simulink model "main_RI_LIEKF"  (R2023a)
settings: Solver=FixedStepAuto  StartTime=0.0  StopTime=220  FixedStep=0.01  RelTol=1e-3
InitFcn:
  | initNavigation0612_AOA;
values from neighbouring files (symbols this model uses):
  CF_enable = 0    [initNavigation.m]
  dt = 0.01    [initNavigation.m]
  dtDelay = -0.03    [initNavigation.m]
  g0 = 9.795    [initNavigation.m]
  gam0_rad = 0/57.3    (= 0)    [initNavigation.m]
  H_sensor_type = 0    [initNavigation.m]
  KF_enable = 1    [initNavigation.m]
  P0 = diag([1*ones(3,1);0.01*ones(3,1);0.1*ones(3,1);0.001*ones(3,1);0.00001*ones(3,1)])    [initNavigation.m]
  P0_RIEKF = diag([1*ones(3,1);0.01*ones(3,1);0.1*ones(3,1);0.001*ones(3,1);0.00001*ones(3,1);      0.01*ones(3,1);[0;2;2]/57.3;[0.1;0.1;0.1]])^2    [initNavigation.m]
  pd0 = 0    [initNavigation.m]
  pe0 = 0    [initNavigation.m]
  phi0_rad = 0/57.3    (= 0)    [initNavigation.m]
  pn0 = 0    [initNavigation.m]
  psi = -178    [initNavigation.m]
  psi0_rad = 0/57.3    (= 0)    [initNavigation.m]
  state_dim = 24    [initNavigation.m]
  Time = 0:0.01:(size(traindata.AttackAngle,1) - 1)*0.01    [NNLiftCoefficientFit.m]
  vd0 = 0    [initNavigation.m]
  ve0 = 0    [initNavigation.m]
  vn0 = 0    [initNavigation.m]
undefined symbols (not defined in the file or in its folder): DiscIntNeverNeededParam, Discrete, INS_CONST, INS_EXPORT, INS_PARAM, magnitude, p, param, pInitialization, sys
libraries: simulink x69, simulink_extras x64, dspstat3 x56, sharedtransform x49, ctrlSharedLib x36, sharedTrackingLibrary x17, FMT_Model_Lib x13, matrix_library x12, deeplib x4, dspsolvers x4, vrlib x4, aerolibconvert2 x1
(part 17 of 22)

== system main_RI_LIEKF/State estimation/distribute CF/distribute CF/Correct/Attitude_Correction/Attitude_Correct ==
  Sensor_Data : Inport
  Rotation_Data : Inport  Port=2
  Acc_Correct : Subsystem
  Subsystem2 : Subsystem
  att_corr_O : Outport
  wires:
  Subsystem2/2(acc_meas_O_mPs2) -> Acc_Correct/2(acc_meas_O_mPs2)  "GPS-加速度估计"
  Acc_Correct/1(att_correct) -> att_corr_O/1
  Subsystem2/3(acc_est_O_mPs2) -> Acc_Correct/3(acc_est_O_mPs2)  "加计-加速度"
  Subsystem2/1(acc_meas_valid) -> Acc_Correct/1(acc_meas_valid)  "GPS状态判断"
  Sensor_Data/1 -> Subsystem2/1(Sensor_Data)
  Rotation_Data/1 -> Subsystem2/2(Rotation_Data)

== system main_RI_LIEKF/State estimation/distribute CF/distribute CF/Correct/Attitude_Correction/Mag_Correct ==
  Rotation_Data : Inport
  Sensor_Data : Inport  Port=2
  Bus Selector1 : BusSelector  OutputSignals=MAGN_Data.mag_norm_B,MAGN_Data.mag_quality
  Bus Selector4 : BusSelector  OutputSignals=M_OB
  MX Product3 : Product  Inputs=3  RndMeth=Simplest
  MX Product4 : Product  Multiplication=Matrix(*)  RndMeth=Simplest
  Relay1 : Relay  OnSwitchValue=0.3  OffSwitchValue=0.2
  Selector4 : Selector  NumberOfDimensions=2  InputPortWidth=3  IndexOptions=Index vector (dialog),Index vector (dialog)  Indices=[2],[1 2 3]  OutputSizes=1,1
  Z axis : Constant  Value=[0 0 1]  OutDataTypeStr=single
  mag_correct_gain : Gain  Gain=MAG_GAIN  OutDataTypeStr=Inherit: Same as input
  mag_corr_O : Outport  VectorParamsAs1DForOutWhenUnconnected=off
  wires:
  Bus Selector4/1 -> Selector4/1  "<M_OB>"
  Rotation_Data/1 -> Bus Selector4/1
  Bus Selector1/2 -> Relay1/1  "<mag_quality>"
  Sensor_Data/1 -> Bus Selector1/1
  mag_correct_gain/1 -> MX Product3/2
  MX Product4/1 -> mag_correct_gain/1  "my_O"
  Selector4/1 -> MX Product4/1
  Relay1/1 -> MX Product3/3  "mag_enable"
  MX Product3/1 -> mag_corr_O/1
  Bus Selector1/1 -> MX Product4/2  "<mag_norm_B>"
  Z axis/1 -> MX Product3/1

== system main_RI_LIEKF/State estimation/distribute CF/distribute CF/Correct/Subsystem2/norm ==
  In1 : Inport
  Sqrt : Sqrt
  Square : Math  Operator=square  SignedPower=on
  Sum of Elements : Sum  Inputs=+
  Out1 : Outport
  wires:
  Sum of Elements/1 -> Sqrt/1
  Square/1 -> Sum of Elements/1
  Sqrt/1 -> Out1/1
  In1/1 -> Square/1

== system main_RI_LIEKF/State estimation/distribute CF/distribute CF/Correct/Subsystem2/低通滤波 ==
  u : Inport
  Constant : Constant  Value=0
  Discrete-Time Integrator : DiscreteIntegrator  ExternalReset=level  SampleTime=-1  ICPrevOutput=DiscIntNeverNeededParam  ICPrevScaledInput=DiscIntNeverNeededParam
  Discrete-Time Integrator1 : DiscreteIntegrator  ExternalReset=level  InitialConditionSource=external  SampleTime=-1  ICPrevOutput=DiscIntNeverNeededParam  ICPrevScaledInput=DiscIntNeverNeededParam
  Gain : Gain  Gain=(2*pi*fc)^2
  Gain1 : Gain  Gain=2*zeta*(2*pi*fc)
  Sum : Sum  Inputs=|+-
  Sum1 : Sum  Inputs=|+-
  y : Outport
  wires:
  Sum/1 -> Gain/1
  Discrete-Time Integrator1/1 -> y/1, Sum/2
  Discrete-Time Integrator/1 -> Gain1/1, Discrete-Time Integrator1/1
  Sum1/1 -> Discrete-Time Integrator/1
  Constant/1 -> Discrete-Time Integrator1/2, Discrete-Time Integrator/2
  u/1 -> Discrete-Time Integrator1/3, Sum/1
  Gain1/1 -> Sum1/2
  Gain/1 -> Sum1/1

== system main_RI_LIEKF/State estimation/distribute CF/distribute CF/Translation_estimate/Rxy_Horizontal_estimation/Integrator_R_Horizontal ==
  Vn : Inport
  dR : Inport  Port=2
  Sensor_data2 : Inport  Port=3
  Cbn : Inport  Port=4
  Add : Sum
  Bus Selector : BusSelector  OutputSignals=QGC_sensor_reinit,GPS_Data.pos_N_gps,GPS_Data.pos_E_gps
  Constant : Constant  Value=[-0.45;0;0]  OutDataTypeStr=single
  Delay : Delay  DelayLength=1  InitialConditionSource=Input port  ExternalReset=Rising
      settings: InputPortMap=u0,r5,p4
  Gain : Gain  Gain=0.1
  Gain2 : Gain  Gain=dt  SaturateOnIntegerOverflow=on  OutDataTypeStr=Inherit: Same as input  ParamDataTypeStr=Inherit: Same as input
  Mux : Mux  Inputs=2
  Product : Product  Multiplication=Matrix(*)
  Selector : Selector  InputPortWidth=3  IndexOptions=Index vector (dialog)  Indices=[1 2]  OutputSizes=1
  Sum : Sum  Inputs=|++-
  R_n&e : Outport
  R_n&eL : Outport  Port=2
  wires:
  dR/1 -> Gain/1
  Vn/1 -> Gain2/1
  Gain2/1 -> Sum/1
  Sensor_data2/1 -> Bus Selector/1
  Bus Selector/1 -> Delay/2  "<QGC_sensor_reinit>"
  Bus Selector/2 -> Mux/1  "<pos_N_gps>"
  Bus Selector/3 -> Mux/2  "<pos_E_gps>"
  Mux/1 -> Delay/3
  Delay/1 -> Sum/2
  Gain/1 -> Sum/3
  Constant/1 -> Product/2
  Product/1 -> Selector/1
  Cbn/1 -> Product/1
  Sum/1 -> Add/1, R_n&e/1, Delay/1
  Selector/1 -> Add/2
  Add/1 -> R_n&eL/1

== system main_RI_LIEKF/State estimation/distribute CF/distribute CF/Translation_estimate/Rxy_Horizontal_estimation/Rxy_kalman filter2 ==
  X : Inport
  Z : Inport  Port=2
  Enable : Inport  Port=3
  Constant : Constant  Value=F  OutDataTypeStr=single
  Constant1 : Constant  Value=Q  OutDataTypeStr=single
  Constant2 : Constant  Value=R  OutDataTypeStr=single
  Constant3 : Constant  Value=P0  OutDataTypeStr=single
  Constant4 : Constant  Value=H  OutDataTypeStr=single
  Vxy kalman filter : Subsystem  TreatAsAtomicUnit=on
  XOut : Outport
  wires:
  Enable/1 -> Vxy kalman filter/9(Enable)
  Vxy kalman filter/1(XOut) -> XOut/1
  Constant1/1 -> Vxy kalman filter/5(Q)
  Constant4/1 -> Vxy kalman filter/4(H)
  Constant2/1 -> Vxy kalman filter/6(R)
  Constant3/1 -> Vxy kalman filter/8(P0)
  Z/1 -> Vxy kalman filter/1(Z)
  Constant/1 -> Vxy kalman filter/3(G), Vxy kalman filter/2(F)
  X/1 -> Vxy kalman filter/7(X)

== system main_RI_LIEKF/State estimation/distribute CF/distribute CF/Translation_estimate/Rxy_Horizontal_estimation/Subsystem ==
  Detect Change1 : simulink/Logic and Bit Operations/Detect Change  vinit=0  InputProcessing=Columns as channels (frame based)  OutDataTypeStr=boolean
  From Workspace1 : FromWorkspace  VariableName=[All.t',All.lat]
  flag : Outport
  wires:
  Detect Change1/1 -> flag/1
  From Workspace1/1 -> Detect Change1/1  "lat"

== system main_RI_LIEKF/State estimation/distribute CF/distribute CF/Translation_estimate/V_Horizontal_estimation/Integrator_V_Horizontal ==
  An : Inport
  dv : Inport  Port=2
  Sensor_data2 : Inport  Port=3
  Bus Selector : BusSelector  OutputSignals=QGC_sensor_reinit,GPS_Data.vn_gps,GPS_Data.ve_gps
  Delay : Delay  DelayLength=1  InitialConditionSource=Input port  ExternalReset=Rising
      settings: InputPortMap=u0,r5,p4
  Gain : Gain
  Gain2 : Gain  Gain=dt  SaturateOnIntegerOverflow=on  OutDataTypeStr=Inherit: Same as input  ParamDataTypeStr=Inherit: Same as input
  Mux : Mux  Inputs=2
  Scope : Scope
  Sum : Sum  Inputs=|++-
  V_n&e : Outport
  wires:
  Gain/1 -> Sum/3, Scope/1
  dv/1 -> Gain/1
  Delay/1 -> Sum/2
  Mux/1 -> Delay/3
  Bus Selector/3 -> Mux/2  "<ve_gps>"
  Bus Selector/2 -> Mux/1  "<vn_gps>"
  Bus Selector/1 -> Delay/2  "<QGC_sensor_reinit>"
  Sensor_data2/1 -> Bus Selector/1
  Sum/1 -> Delay/1, V_n&e/1
  Gain2/1 -> Sum/1
  An/1 -> Gain2/1

== system main_RI_LIEKF/State estimation/distribute CF/distribute CF/Translation_estimate/V_Horizontal_estimation/Rxy_kalman filter1 ==
  X : Inport
  Z : Inport  Port=2
  Enable : Inport  Port=3
  Constant : Constant  Value=F  OutDataTypeStr=single
  Constant1 : Constant  Value=Q  OutDataTypeStr=single
  Constant2 : Constant  Value=R  OutDataTypeStr=single
  Constant3 : Constant  Value=P0  OutDataTypeStr=single
  Constant4 : Constant  Value=H  OutDataTypeStr=single
  Vxy kalman filter : Subsystem  TreatAsAtomicUnit=on
  XOut : Outport
  wires:
  X/1 -> Vxy kalman filter/7(X)
  Constant/1 -> Vxy kalman filter/2(F), Vxy kalman filter/3(G)
  Z/1 -> Vxy kalman filter/1(Z)
  Constant3/1 -> Vxy kalman filter/8(P0)
  Constant2/1 -> Vxy kalman filter/6(R)
  Constant4/1 -> Vxy kalman filter/4(H)
  Constant1/1 -> Vxy kalman filter/5(Q)
  Vxy kalman filter/1(XOut) -> XOut/1
  Enable/1 -> Vxy kalman filter/9(Enable)

== system main_RI_LIEKF/State estimation/distribute CF/distribute CF/Update/Attitude_Update/uniformization1 ==
  Q i : Inport  PortDimensions=4
  Constant : Constant  Value=1e-20
  Dot Product1 : DotProduct  OutDataTypeStr=Inherit: Inherit via internal rule
  Math Function : Math  Operator=sqrt  SignedPower=on
  Product : Product  Inputs=*/  SaturateOnIntegerOverflow=on  OutDataTypeStr=Inherit: Same as first input
  Sum : Sum  Inputs=|++  SaturateOnIntegerOverflow=on
  Q o : Outport
  wires:
  Sum/1 -> Product/2
  Constant/1 -> Sum/2
  Product/1 -> Q o/1
  Math Function/1 -> Sum/1
  Dot Product1/1 -> Math Function/1
  Q i/1 -> Product/1, Dot Product1/1, Dot Product1/2

== system main_RI_LIEKF/State estimation/distribute CF/distribute CF/初始化/Attitude_Reset/Reset Heading ==
  note: When GPS is valid at first time, the mag data will be compensated with WMM data,
      | so we need reset attitude.
  GPS_valid : Inport
  Add : Sum  AccumDataTypeStr=uint32
  Compare To Constant : simulink/Logic and Bit Operations/Compare To Constant  relop=>=  const=1  OutDataTypeStr=boolean
  Data Type Conversion : DataTypeConversion  OutDataTypeStr=uint32  SaturateOnIntegerOverflow=off  RndMeth=Floor
  Delay : Delay  DelayLength=1
  Detect Rise Positive1 : simulink/Logic and Bit Operations/Detect Rise Positive  vinit=0  OutDataTypeStr=boolean
  Saturation : Saturate  UpperLimit=1  LowerLimit=0
  reset : Outport
  wires:
  Delay/1 -> Add/2
  Data Type Conversion/1 -> Add/1
  GPS_valid/1 -> Compare To Constant/1
  Detect Rise Positive1/1 -> reset/1
  Add/1 -> Saturation/1
  Saturation/1 -> Detect Rise Positive1/1, Delay/1
  Compare To Constant/1 -> Data Type Conversion/1

== system main_RI_LIEKF/State estimation/distribute CF/distribute CF/初始化/Attitude_Reset/norm ==
  In1 : Inport
  Sqrt : Sqrt
  Square : Math  Operator=square  SignedPower=on
  Sum of Elements : Sum  Inputs=+
  Out1 : Outport
  wires:
  Sum of Elements/1 -> Sqrt/1
  Square/1 -> Sum of Elements/1
  Sqrt/1 -> Out1/1
  In1/1 -> Square/1

== system main_RI_LIEKF/State estimation/distribute CF/distribute CF/初始化/Attitude_Reset/sample_valid ==
  valid : Inport
  Add : Sum  AccumDataTypeStr=uint32
  Data Type Conversion : DataTypeConversion  OutDataTypeStr=uint32  SaturateOnIntegerOverflow=off  RndMeth=Floor
  Delay : Delay  DelayLength=1
  Saturation : Saturate  UpperLimit=10000  LowerLimit=0
  valid_samples : simulink/Logic and Bit Operations/Compare To Constant  relop=>  const=50  OutDataTypeStr=boolean
  sample_valid : Outport
  wires:
  Add/1 -> Saturation/1
  valid_samples/1 -> sample_valid/1
  Delay/1 -> Add/2
  valid/1 -> Data Type Conversion/1
  Data Type Conversion/1 -> Add/1
  Saturation/1 -> valid_samples/1, Delay/1

== system main_RI_LIEKF/State estimation/distribute CF/distribute CF/初始化/Subsystem/Normalized1 ==
  fb : Inport
  Add : Sum
  Constant : Constant  Value=1e-6  OutDataTypeStr=single
  Divide : Product  Inputs=*/
  Math Function : Math  Operator=magnitude^2  SignedPower=on
  Sqrt : Sqrt
  Sum of Elements : Sum  Inputs=+
  fb/g : Outport
  wires:
  Math Function/1 -> Sum of Elements/1
  Divide/1 -> fb/g/1
  Sum of Elements/1 -> Sqrt/1
  fb/1 -> Divide/1, Math Function/1
  Add/1 -> Divide/2
  Sqrt/1 -> Add/1
  Constant/1 -> Add/2

== system main_RI_LIEKF/State estimation/distribute CF/distribute CF/初始化/Subsystem/Normalized2 ==
  fb : Inport
  Add : Sum
  Constant : Constant  Value=1e-6  OutDataTypeStr=single
  Divide : Product  Inputs=*/
  Math Function : Math  Operator=magnitude^2  SignedPower=on
  Sqrt : Sqrt
  Sum of Elements : Sum  Inputs=+
  fb/g : Outport
  wires:
  Math Function/1 -> Sum of Elements/1
  Divide/1 -> fb/g/1
  Sum of Elements/1 -> Sqrt/1
  fb/1 -> Divide/1, Math Function/1
  Add/1 -> Divide/2
  Sqrt/1 -> Add/1
  Constant/1 -> Add/2

== system main_RI_LIEKF/State estimation/distribute CF/distribute CF/初始化/Subsystem/Normalized3 ==
  fb : Inport
  Add : Sum
  Constant : Constant  Value=1e-6  OutDataTypeStr=single
  Divide : Product  Inputs=*/
  Math Function : Math  Operator=magnitude^2  SignedPower=on
  Sqrt : Sqrt
  Sum of Elements : Sum  Inputs=+
  fb/g : Outport
  wires:
  Math Function/1 -> Sum of Elements/1
  Divide/1 -> fb/g/1
  Sum of Elements/1 -> Sqrt/1
  fb/1 -> Divide/1, Math Function/1
  Add/1 -> Divide/2
  Sqrt/1 -> Add/1
  Constant/1 -> Add/2

== system main_RI_LIEKF/Sensor_Data_Process/Magn_Data_Process1/Mag_Data_Process/Mag_Quality_Estimate/Mag_Quality/Inclination_Quality_Estimate/Norm(x) ==
  In1 : Inport
  Sqrt : Sqrt
  Square : Math  Operator=square  SignedPower=on
  Sum of Elements : Sum  Inputs=+
  Out1 : Outport
  wires:
  In1/1 -> Square/1
  Sqrt/1 -> Out1/1
  Sum of Elements/1 -> Sqrt/1
  Square/1 -> Sum of Elements/1

== system main_RI_LIEKF/Sensor_Data_Process/Magn_Data_Process1/Mag_Data_Process/Mag_Quality_Estimate/Mag_Quality/Intensity_Quality_Estimate/Norm(x) ==
  In1 : Inport
  Sqrt : Sqrt
  Square : Math  Operator=square  SignedPower=on
  Sum of Elements : Sum  Inputs=+
  Out1 : Outport
  wires:
  Sum of Elements/1 -> Sqrt/1
  Square/1 -> Sum of Elements/1
  Sqrt/1 -> Out1/1
  In1/1 -> Square/1

== system main_RI_LIEKF/State estimation/distribute CF/Translation_estimate/Rxy_Horizontal_estimation/Rxy_kalman filter2/Vxy kalman filter/kalman ==
  note: Xk/k-1=FXk-1
      | Xk=Xk/k-1+K(Z-h(Xk/k-1))
      | K=Pk/k-1H(HPk/k-1H+Rk)-1
      | Pk/k-1=FPk-1F+GQG
      | Pk=(I-KH)Pk/k-1
  Z : Inport
  F : Inport  Port=2
  G : Inport  Port=3
  H : Inport  Port=4
  Q : Inport  Port=5
  R : Inport  Port=6
  P : Inport  Port=7
  X : Inport  Port=8
  Enable : Inport  Port=9
  Subsystem : Subsystem
  Subsystem1 : Subsystem
  POut : Outport
  XOut : Outport  Port=2
  wires:
  X/1 -> [X]
  P/1 -> [P]
  Q/1 -> [Q]
  G/1 -> [G]
  F/1 -> [F]
  Z/1 -> [Z]
  [F] -> Subsystem/1(F)
  [G] -> Subsystem/2(G)
  [Q] -> Subsystem/3(Q)
  [X] -> Subsystem/4(X)
  [P] -> Subsystem/5(P)
  Subsystem/1(Xk_k_1) -> [Xk_k_1]
  Subsystem/2(Pk_k_1) -> [Pk_k_1]
  H/1 -> Subsystem1/3(H)
  R/1 -> Subsystem1/4(R)
  Subsystem1/1(POut) -> POut/1
  Subsystem1/2(XOut) -> XOut/1
  [Xk_k_1] -> Subsystem1/1(Xkk)
  [Pk_k_1] -> Subsystem1/2(Pkk)
  Enable/1 -> Subsystem1/Enable
  [Z] -> Subsystem1/5(Z)

== system main_RI_LIEKF/State estimation/distribute CF/Translation_estimate/V_Horizontal_estimation/Rxy_kalman filter1/Vxy kalman filter/kalman ==
  note: Xk/k-1=FXk-1
      | Xk=Xk/k-1+K(Z-h(Xk/k-1))
      | K=Pk/k-1H(HPk/k-1H+Rk)-1
      | Pk/k-1=FPk-1F+GQG
      | Pk=(I-KH)Pk/k-1
  Z : Inport
  F : Inport  Port=2
  G : Inport  Port=3
  H : Inport  Port=4
  Q : Inport  Port=5
  R : Inport  Port=6
  P : Inport  Port=7
  X : Inport  Port=8
  Enable : Inport  Port=9
  Scope : Scope  NumInputPorts=2
  Subsystem : Subsystem
  Subsystem1 : Subsystem
  POut : Outport
  XOut : Outport  Port=2
  wires:
  [Z] -> Subsystem1/5(Z)
  Enable/1 -> Scope/1, Subsystem1/Enable
  [Pk_k_1] -> Subsystem1/2(Pkk)
  [Xk_k_1] -> Subsystem1/1(Xkk)
  Subsystem1/2(XOut) -> Scope/2, XOut/1
  Subsystem1/1(POut) -> POut/1
  R/1 -> Subsystem1/4(R)
  H/1 -> Subsystem1/3(H)
  Subsystem/2(Pk_k_1) -> [Pk_k_1]
  Subsystem/1(Xk_k_1) -> [Xk_k_1]
  [P] -> Subsystem/5(P)
  [X] -> Subsystem/4(X)
  [Q] -> Subsystem/3(Q)
  [G] -> Subsystem/2(G)
  [F] -> Subsystem/1(F)
  Z/1 -> [Z]
  F/1 -> [F]
  G/1 -> [G]
  Q/1 -> [Q]
  P/1 -> [P]
  X/1 -> [X]

== system main_RI_LIEKF/State estimation/distribute CF/distribute CF/AHRS1/Correct/Attitude_Correction/Attitude_Correct ==
  Rotation_Data : Inport
  Sensor_Data : Inport  Port=2
  Acc_Correct : Subsystem
  Acc_Estimator : Subsystem
  att_corr_O : Outport
  wires:
  Acc_Estimator/3(acc_est_O_mPs2) -> Acc_Correct/3(acc_est_O_mPs2)  "acc_est_O_mPs2"
  Sensor_Data/1 -> Acc_Estimator/1(Sensor_Data)
  Rotation_Data/1 -> Acc_Estimator/2(Rotation_Data)
  Acc_Correct/1(att_correct) -> att_corr_O/1
  Acc_Estimator/1(acc_meas_valid) -> Acc_Correct/1(acc_meas_valid)  "acc_meas_valid"
  Acc_Estimator/2(acc_meas_O_mPs2) -> Acc_Correct/2(acc_meas_O_mPs2)  "acc_meas_O_mPs2"

== system main_RI_LIEKF/State estimation/distribute CF/distribute CF/AHRS1/Correct/Attitude_Correction/Mag_Correct ==
  Rotation_Data : Inport
  Sensor_Data : Inport  Port=2
  standstill : Inport  Port=3
  Bus Selector1 : BusSelector  OutputSignals=Mag_Data.mag_norm_B,Mag_Data.mag_quality
  Bus Selector4 : BusSelector  OutputSignals=M_OB
  Constant : Constant  Value=INS_PARAM.MAG_AIR_EN
  Logical Operator : Logic  AllPortsSameDT=off  OutDataTypeStr=boolean
  Logical Operator1 : Logic  Operator=OR  AllPortsSameDT=off  OutDataTypeStr=boolean
  MX Product3 : Product  Inputs=3  RndMeth=Simplest
  MX Product4 : Product  Multiplication=Matrix(*)  RndMeth=Simplest
  Relay1 : Relay  OnSwitchValue=0.3  OffSwitchValue=0.2
  Selector4 : Selector  NumberOfDimensions=2  InputPortWidth=3  IndexOptions=Index vector (dialog),Index vector (dialog)  Indices=[2],[1 2 3]  OutputSizes=1,1
  Subsystem : Subsystem  Commented=on
  Z axis : Constant  Value=[0 0 1]  OutDataTypeStr=single
  mag_correct_gain : Gain  Gain=-INS_PARAM.MAG_GAIN  OutDataTypeStr=Inherit: Same as input
  mag_corr_O : Outport
  wires:
  Bus Selector4/1 -> Subsystem/1(M_OB), Selector4/1  "<M_OB>"
  Rotation_Data/1 -> Subsystem/3(Rotation_Data), Bus Selector4/1
  Bus Selector1/2 -> Relay1/1  "<mag_quality>"
  Sensor_Data/1 -> Bus Selector1/1
  mag_correct_gain/1 -> MX Product3/2
  MX Product4/1 -> mag_correct_gain/1  "my_O"
  Selector4/1 -> MX Product4/1
  Relay1/1 -> Logical Operator/1  "mag_enable"
  Logical Operator/1 -> MX Product3/3
  Logical Operator1/1 -> Logical Operator/2
  Constant/1 -> Logical Operator1/1
  standstill/1 -> Logical Operator1/2
  MX Product3/1 -> mag_corr_O/1
  Bus Selector1/1 -> Subsystem/2(mag_B), MX Product4/2  "<mag_norm_B>"
  Z axis/1 -> MX Product3/1

== system main_RI_LIEKF/State estimation/distribute CF/distribute CF/Correct/Attitude_Correction/Attitude_Correct/Acc_Correct ==
  note: 加计的加速度
      | &
      | GPS的加速度估计
  acc_meas_valid : Inport
  acc_meas_O_mPs2 : Inport  Port=2
  acc_est_O_mPs2 : Inport  Port=3
  Heading_Correct : Subsystem
  Scope : Scope  NumInputPorts=2
  Sum : Sum  Inputs=|++
  Verticle_Correct : Subsystem
  att_correct : Outport
  wires:
  acc_meas_valid/1 -> Heading_Correct/3(acc_meas_valid)
  Verticle_Correct/1(vert_correct) -> Sum/1  "vert_correct"
  Heading_Correct/1(heading_correct) -> Sum/2, Scope/2  "heading_correct"
  acc_meas_O_mPs2/1 -> Verticle_Correct/2(acc_meas_O_mPs2), Heading_Correct/2(acc_meas_O_mPs2)
  acc_est_O_mPs2/1 -> Verticle_Correct/1(acc_est_O_mPs2), Heading_Correct/1(acc_est_O_mPs2)
  Sum/1 -> Scope/1, att_correct/1

== system main_RI_LIEKF/State estimation/distribute CF/distribute CF/Correct/Attitude_Correction/Attitude_Correct/Subsystem2 ==
  Sensor_Data : Inport
  Rotation_Data : Inport  Port=2
  Bus Selector : BusSelector  OutputSignals=GPS_Data.vn_gps,GPS_Data.ve_gps,GPS_Data.vd_gps
  Data Type Conversion : DataTypeConversion  OutDataTypeStr=single  SaturateOnIntegerOverflow=off  RndMeth=Floor
  Estimate_Acc : Subsystem
  MATLAB Function : MATLAB Function  TreatAsAtomicUnit=on
  Math Function : Math  Operator=magnitude^2  SignedPower=on
  Multiply : Product  OutDataTypeStr=single
  Mux : Mux  Inputs=3
  Scope : Scope
  Scope1 : Scope  NumInputPorts=2
  Scope2 : Scope  NumInputPorts=2
  Sqrt : Sqrt
  Sum of Elements : Sum  Inputs=+
  Sum2 : Sum  Inputs=++|
  gps_meas_acc-加速度估计 : Subsystem
  gravity-an : Constant  Value=[0;0;-g0]  VectorParams1D=off  OutDataTypeStr=single
  acc_meas_valid : Outport
  acc_meas_O_mPs2 : Outport  Port=2
  acc_est_O_mPs2 : Outport  Port=3
  wires:
  Sum2/1 -> Scope1/1, acc_meas_O_mPs2/1
  gps_meas_acc-加速度估计/1(gps_meas_valid) -> Scope/1, Estimate_Acc/1(gps_meas_valid), acc_meas_valid/1, Multiply/1
  gps_meas_acc-加速度估计/2(gps_meas_acc) -> Multiply/2
  MATLAB Function/1(y) -> Data Type Conversion/1
  Rotation_Data/1 -> Estimate_Acc/3(Rotation_Data)
  Estimate_Acc/1(加计-加速度估计acc_est_O_mPs2) -> Scope1/2, acc_est_O_mPs2/1
  gravity-an/1 -> Sum2/1
  Sensor_Data/1 -> Estimate_Acc/2(Sensor_Data), gps_meas_acc-加速度估计/1(Sensor_Data), Bus Selector/1
  Math Function/1 -> Sum of Elements/1
  Bus Selector/1 -> Mux/1  "<vn_gps>"
  Bus Selector/2 -> Mux/2  "<ve_gps>"
  Mux/1 -> Math Function/1
  Sum of Elements/1 -> Sqrt/1
  Sqrt/1 -> Scope2/1, MATLAB Function/1(abs_v)
  Multiply/1 -> Scope2/2, MATLAB Function/2(gps_acc)
  Bus Selector/3 -> Mux/3  "<vd_gps>"
  Data Type Conversion/1 -> Sum2/2

== system main_RI_LIEKF/State estimation/distribute CF/distribute CF/Translation_estimate/Rxy_Horizontal_estimation/Rxy_kalman filter2/Vxy kalman filter ==
  Z : Inport
  F : Inport  Port=2
  G : Inport  Port=3
  H : Inport  Port=4
  Q : Inport  Port=5
  R : Inport  Port=6
  X : Inport  Port=7
  P0 : Inport  Port=8
  Enable : Inport  Port=9
  Add1 : Sum
  Delay : Delay  DelayLength=1  InitialConditionSource=Input port
      settings: InputPortMap=u0,p4
  Gain4 : Gain  Gain=0.5
  Math Function : Math  Operator=transpose  SignedPower=on
  kalman : Subsystem
  XOut : Outport
  wires:
  P0/1 -> Delay/2
  Gain4/1 -> Delay/1
  Delay/1 -> kalman/7(P)
  Add1/1 -> Gain4/1
  Math Function/1 -> Add1/2
  Z/1 -> kalman/1(Z)
  F/1 -> kalman/2(F)
  G/1 -> kalman/3(G)
  H/1 -> kalman/4(H)
  Q/1 -> kalman/5(Q)
  R/1 -> kalman/6(R)
  X/1 -> kalman/8(X)
  kalman/1(POut) -> Math Function/1, Add1/1
  kalman/2(XOut) -> XOut/1
  Enable/1 -> kalman/9(Enable)

== system main_RI_LIEKF/State estimation/distribute CF/distribute CF/Translation_estimate/V_Horizontal_estimation/Rxy_kalman filter1/Vxy kalman filter ==
  Z : Inport
  F : Inport  Port=2
  G : Inport  Port=3
  H : Inport  Port=4
  Q : Inport  Port=5
  R : Inport  Port=6
  X : Inport  Port=7
  P0 : Inport  Port=8
  Enable : Inport  Port=9
  Add1 : Sum
  Delay : Delay  DelayLength=1  InitialConditionSource=Input port
      settings: InputPortMap=u0,p4
  Gain4 : Gain  Gain=0.5
  Math Function : Math  Operator=transpose  SignedPower=on
  kalman : Subsystem
  XOut : Outport
  wires:
  Enable/1 -> kalman/9(Enable)
  kalman/2(XOut) -> XOut/1
  kalman/1(POut) -> Add1/1, Math Function/1
  X/1 -> kalman/8(X)
  R/1 -> kalman/6(R)
  Q/1 -> kalman/5(Q)
  H/1 -> kalman/4(H)
  G/1 -> kalman/3(G)
  F/1 -> kalman/2(F)
  Z/1 -> kalman/1(Z)
  Math Function/1 -> Add1/2
  Add1/1 -> Gain4/1
  Delay/1 -> kalman/7(P)
  Gain4/1 -> Delay/1
  P0/1 -> Delay/2

== system main_RI_LIEKF/State estimation/distribute CF/Translation_estimate/Rxy_Horizontal_estimation/Rxy_kalman filter2/Vxy kalman filter/kalman/Subsystem ==
  F : Inport
  G : Inport  Port=2
  Q : Inport  Port=3
  X : Inport  Port=4
  P : Inport  Port=5
  Add : Sum
  Math Function3 : Math  Operator=transpose  SignedPower=on
  Math Function4 : Math  Operator=transpose  SignedPower=on
  MatrixMultiply : Product  Multiplication=Matrix(*)
  MatrixMultiply1 : Product  Inputs=3  Multiplication=Matrix(*)
  MatrixMultiply8 : Product  Inputs=3  Multiplication=Matrix(*)
  Xk_k_1 : Outport
  Pk_k_1 : Outport  Port=2
  wires:
  Math Function4/1 -> MatrixMultiply8/3
  [Q] -> MatrixMultiply8/2
  MatrixMultiply/1 -> [Xk_k_1]
  MatrixMultiply1/1 -> Add/1
  [F] -> Math Function3/1
  Math Function3/1 -> MatrixMultiply1/3
  [P] -> MatrixMultiply1/2
  [F] -> MatrixMultiply1/1
  Add/1 -> [Pk_k_1]
  [G] -> MatrixMultiply8/1
  MatrixMultiply8/1 -> Add/2
  [X] -> MatrixMultiply/2
  [G] -> Math Function4/1
  [F] -> MatrixMultiply/1
  F/1 -> [F]
  G/1 -> [G]
  Q/1 -> [Q]
  X/1 -> [X]
  P/1 -> [P]
  [Xk_k_1] -> Xk_k_1/1
  [Pk_k_1] -> Pk_k_1/1

== system main_RI_LIEKF/State estimation/distribute CF/Translation_estimate/Rxy_Horizontal_estimation/Rxy_kalman filter2/Vxy kalman filter/kalman/Subsystem1 ==
  note: 计算卡尔曼增益Kk
  Xkk : Inport
  Pkk : Inport  Port=2
  H : Inport  Port=3
  R : Inport  Port=4
  Z : Inport  Port=5
  Enable : EnablePort
  Add2 : Sum
  Add3 : Sum  Inputs=+-
  Add4 : Sum  Inputs=+-
  Add5 : Sum
  Constant : Constant  Value=eye(4)  OutDataTypeStr=single
  LDL Solver1 : dspsolvers/LDL Solver  errmode=Warning
      settings: RTWMemSecFuncInitTerm=Default  RTWMemSecFuncExecute=Default  RTWMemSecDataConstants=Default  RTWMemSecDataInternal=Default  RTWMemSecDataParameters=Default
  Math Function5 : Math  Operator=transpose  SignedPower=on
  Math Function6 : Math  Operator=transpose  SignedPower=on
  MatrixMultiply{4..7,9..10} (6 alike) : Product  Multiplication=Matrix(*)
  Scope : Scope
  POut : Outport
  XOut : Outport  Port=2
  wires:
  MatrixMultiply9/1 -> Add3/2
  MatrixMultiply7/1 -> POut/1
  [H] -> MatrixMultiply10/1
  Add3/1 -> MatrixMultiply4/2
  Math Function5/1 -> MatrixMultiply5/2
  Math Function6/1 -> Scope/1, [Kk]
  Add4/1 -> MatrixMultiply7/1
  MatrixMultiply4/1 -> Add2/2
  [Kk] -> MatrixMultiply4/1
  [Z] -> Add3/1
  MatrixMultiply10/1 -> MatrixMultiply5/1, LDL Solver1/2
  MatrixMultiply5/1 -> Add5/1
  LDL Solver1/1 -> Math Function6/1
  [H] -> Math Function5/1
  [Pk_k_1] -> MatrixMultiply10/2
  [R] -> Add5/2
  Constant/1 -> Add4/1
  [Kk] -> MatrixMultiply6/1
  [Xk_k_1] -> Add2/1
  [H] -> MatrixMultiply6/2
  [H] -> MatrixMultiply9/1
  [Xk_k_1] -> MatrixMultiply9/2
  [Pk_k_1] -> MatrixMultiply7/2
  R/1 -> [R]
  Add5/1 -> LDL Solver1/1
  MatrixMultiply6/1 -> Add4/2
  H/1 -> [H]
  Add2/1 -> XOut/1
  Xkk/1 -> [Xk_k_1]
  Z/1 -> [Z]
  Pkk/1 -> [Pk_k_1]

== system main_RI_LIEKF/State estimation/distribute CF/Translation_estimate/V_Horizontal_estimation/Rxy_kalman filter1/Vxy kalman filter/kalman/Subsystem ==
  F : Inport
  G : Inport  Port=2
  Q : Inport  Port=3
  X : Inport  Port=4
  P : Inport  Port=5
  Add : Sum
  Math Function3 : Math  Operator=transpose  SignedPower=on
  Math Function4 : Math  Operator=transpose  SignedPower=on
  MatrixMultiply : Product  Multiplication=Matrix(*)
  MatrixMultiply1 : Product  Inputs=3  Multiplication=Matrix(*)
  MatrixMultiply8 : Product  Inputs=3  Multiplication=Matrix(*)
  Xk_k_1 : Outport
  Pk_k_1 : Outport  Port=2
  wires:
  [Pk_k_1] -> Pk_k_1/1
  [Xk_k_1] -> Xk_k_1/1
  P/1 -> [P]
  X/1 -> [X]
  Q/1 -> [Q]
  G/1 -> [G]
  F/1 -> [F]
  [F] -> MatrixMultiply/1
  [G] -> Math Function4/1
  [X] -> MatrixMultiply/2
  MatrixMultiply8/1 -> Add/2
  [G] -> MatrixMultiply8/1
  Add/1 -> [Pk_k_1]
  [F] -> MatrixMultiply1/1
  [P] -> MatrixMultiply1/2
  Math Function3/1 -> MatrixMultiply1/3
  [F] -> Math Function3/1
  MatrixMultiply1/1 -> Add/1
  MatrixMultiply/1 -> [Xk_k_1]
  [Q] -> MatrixMultiply8/2
  Math Function4/1 -> MatrixMultiply8/3

== system main_RI_LIEKF/State estimation/distribute CF/Translation_estimate/V_Horizontal_estimation/Rxy_kalman filter1/Vxy kalman filter/kalman/Subsystem1 ==
  note: 计算卡尔曼增益Kk
  Xkk : Inport
  Pkk : Inport  Port=2
  H : Inport  Port=3
  R : Inport  Port=4
  Z : Inport  Port=5
  Enable : EnablePort
  Add2 : Sum
  Add3 : Sum  Inputs=+-
  Add4 : Sum  Inputs=+-
  Add5 : Sum
  Constant : Constant  Value=eye(4)  OutDataTypeStr=single
  LDL Solver1 : dspsolvers/LDL Solver  errmode=Warning
      settings: RTWMemSecFuncInitTerm=Default  RTWMemSecFuncExecute=Default  RTWMemSecDataConstants=Default  RTWMemSecDataInternal=Default  RTWMemSecDataParameters=Default
  Math Function5 : Math  Operator=transpose  SignedPower=on
  Math Function6 : Math  Operator=transpose  SignedPower=on
  MatrixMultiply{4..7,9..10} (6 alike) : Product  Multiplication=Matrix(*)
  Scope : Scope
  POut : Outport
  XOut : Outport  Port=2
  wires:
  Pkk/1 -> [Pk_k_1]
  Z/1 -> [Z]
  Xkk/1 -> [Xk_k_1]
  Add2/1 -> XOut/1
  H/1 -> [H]
  MatrixMultiply6/1 -> Add4/2
  Add5/1 -> LDL Solver1/1
  R/1 -> [R]
  [Pk_k_1] -> MatrixMultiply7/2
  [Xk_k_1] -> MatrixMultiply9/2
  [H] -> MatrixMultiply9/1
  [H] -> MatrixMultiply6/2
  [Xk_k_1] -> Add2/1
  [Kk] -> MatrixMultiply6/1
  Constant/1 -> Add4/1
  [R] -> Add5/2
  [Pk_k_1] -> MatrixMultiply10/2
  [H] -> Math Function5/1
  LDL Solver1/1 -> Math Function6/1
  MatrixMultiply5/1 -> Add5/1
  MatrixMultiply10/1 -> LDL Solver1/2, MatrixMultiply5/1
  [Z] -> Add3/1
  [Kk] -> MatrixMultiply4/1
  MatrixMultiply4/1 -> Add2/2
  Add4/1 -> MatrixMultiply7/1
  Math Function6/1 -> [Kk], Scope/1
  Math Function5/1 -> MatrixMultiply5/2
  Add3/1 -> MatrixMultiply4/2
  [H] -> MatrixMultiply10/1
  MatrixMultiply7/1 -> POut/1
  MatrixMultiply9/1 -> Add3/2

== system main_RI_LIEKF/State estimation/distribute CF/distribute CF/AHRS1/Correct/Attitude_Correction/Attitude_Correct/Acc_Correct ==
  acc_meas_valid : Inport
  acc_meas_O_mPs2 : Inport  Port=2
  acc_est_O_mPs2 : Inport  Port=3
  Heading_Correct : Subsystem
  Sum : Sum  Inputs=|++
  Verticle_Correct : Subsystem
  att_correct : Outport
  wires:
  acc_meas_valid/1 -> Heading_Correct/3(acc_meas_valid)
  Verticle_Correct/1(vert_correct) -> Sum/1  "vert_correct"
  Heading_Correct/1(heading_correct) -> Sum/2  "heading_correct"
  acc_meas_O_mPs2/1 -> Verticle_Correct/2(acc_meas_O_mPs2), Heading_Correct/2(acc_meas_O_mPs2)
  acc_est_O_mPs2/1 -> Verticle_Correct/1(acc_est_O_mPs2), Heading_Correct/1(acc_est_O_mPs2)
  Sum/1 -> att_correct/1

== system main_RI_LIEKF/State estimation/distribute CF/distribute CF/AHRS1/Correct/Attitude_Correction/Attitude_Correct/Acc_Estimator ==
  Sensor_Data : Inport
  Rotation_Data : Inport  Port=2
  Estimate_Acc : Subsystem
  Measure_Acc : Subsystem
  Multiply : Product  OutDataTypeStr=single
  Sum2 : Sum  Inputs=++|
  gravity : Constant  Value=[0;0;-INS_CONST.g]  VectorParams1D=off  OutDataTypeStr=single
  acc_meas_valid : Outport
  acc_meas_O_mPs2 : Outport  Port=2
  acc_est_O_mPs2 : Outport  Port=3
  wires:
  Measure_Acc/1(gps_meas_valid) -> Estimate_Acc/1(gps_meas_valid), acc_meas_valid/1, Multiply/1
  Sum2/1 -> acc_meas_O_mPs2/1
  Sensor_Data/1 -> Estimate_Acc/2(Sensor_Data), Measure_Acc/1(Sensor_Data)
  gravity/1 -> Sum2/1
  Multiply/1 -> Sum2/2
  Measure_Acc/2(gps_meas_acc) -> Multiply/2
  Rotation_Data/1 -> Estimate_Acc/3(Rotation_Data)
  Estimate_Acc/1(acc_est_O_mPs2) -> acc_est_O_mPs2/1

== system main_RI_LIEKF/State estimation/distribute CF/distribute CF/AHRS1/Correct/Attitude_Correction/Mag_Correct/Subsystem ==
  M_OB : Inport
  mag_B : Inport  Port=2
  Rotation_Data : Inport  Port=3
  Add : Sum
  Atan2 : Trigonometry  Operator=atan2
  Bus Selector : BusSelector  OutputSignals=psi_rad
  Demux : Demux  Outputs=3
  Gain : Gain  Gain=-1
  MX Product1 : Product  Multiplication=Matrix(*)  RndMeth=Simplest
  Terminator : Terminator
  Terminator1 : Terminator
  wires:
  Demux/3 -> Terminator1/1
  Atan2/1 -> Add/1
  Demux/1 -> Atan2/2
  MX Product1/1 -> Demux/1  "my_O"
  Gain/1 -> Atan2/1
  Add/1 -> Terminator/1  "mag_heading"
  Rotation_Data/1 -> Bus Selector/1
  Bus Selector/1 -> Add/2  "<psi_rad>"
  Demux/2 -> Gain/1
  mag_B/1 -> MX Product1/2
  M_OB/1 -> MX Product1/1

== system main_RI_LIEKF/State estimation/distribute CF/distribute CF/Correct/Attitude_Correction/Attitude_Correct/Acc_Correct/Heading_Correct ==
  acc_est_O_mPs2 : Inport
  acc_meas_O_mPs2 : Inport  Port=2
  acc_meas_valid : Inport  Port=3
  Cross Product1 : vrlib/Utilities/Cross Product
  Dead Zone2 : DeadZone  LowerValue=-0.2  UpperValue=0.2
  Demux : Demux  Outputs=3
  Demux1 : Demux  Outputs=3
  Gain : Gain  Gain=att_heading_correct_gain  OutDataTypeStr=single
  Gain1 : Gain  Gain=0
  Gain2 : Gain  Gain=0
  Multiply : Product
  Mux1 : Mux  Inputs=3
  Mux2 : Mux  Inputs=3
  Saturation : Saturate
  heading_correct : Outport
  wires:
  Dead Zone2/1 -> Gain/1  "test1"
  Saturation/1 -> Multiply/1
  Mux1/1 -> Cross Product1/2
  Cross Product1/1 -> Dead Zone2/1
  Demux/1 -> Mux1/1
  acc_meas_valid/1 -> Multiply/2
  Multiply/1 -> heading_correct/1
  Gain/1 -> Saturation/1
  acc_meas_O_mPs2/1 -> Demux/1
  Demux/2 -> Mux1/2
  Demux/3 -> Gain1/1
  Gain1/1 -> Mux1/3
  Demux1/2 -> Mux2/2
  Mux2/1 -> Cross Product1/1
  Gain2/1 -> Mux2/3
  Demux1/1 -> Mux2/1
  Demux1/3 -> Gain2/1
  acc_est_O_mPs2/1 -> Demux1/1

== system main_RI_LIEKF/State estimation/distribute CF/distribute CF/Correct/Attitude_Correction/Attitude_Correct/Acc_Correct/Verticle_Correct ==
  acc_est_O_mPs2 : Inport
  acc_meas_O_mPs2 : Inport  Port=2
  Cross Product1 : vrlib/Utilities/Cross Product
  Gain1 : Gain  Gain=[att_correct_gain;att_correct_gain;0]
  Normalized : Subsystem
  Normalized1 : Subsystem
  Saturation : Subsystem
  vert_correct : Outport
  wires:
  Cross Product1/1 -> Saturation/1(u)
  Normalized/1(fb/g) -> Cross Product1/1
  acc_meas_O_mPs2/1 -> Normalized1/1(fb)
  Saturation/1(y) -> Gain1/1
  acc_est_O_mPs2/1 -> Normalized/1(fb)
  Normalized1/1(fb/g) -> Cross Product1/2
  Gain1/1 -> vert_correct/1

== system main_RI_LIEKF/State estimation/distribute CF/distribute CF/Correct/Attitude_Correction/Attitude_Correct/Subsystem2/Estimate_Acc ==
  gps_meas_valid : Inport
  Sensor_Data : Inport  Port=2
  Rotation_Data : Inport  Port=3
  Bus Selector : BusSelector  OutputSignals=IMU_Data.accl_B_m/s2_LPF
  Bus Selector1 : BusSelector  OutputSignals=M_OB
  Delay : Delay  DelayLengthSource=Input port  DelayLengthUpperLimit=200
      settings: InputPortMap=u0,p1
  GPS_Delay : Constant  OutDataTypeStr=uint16
  Multiply : Product  Multiplication=Matrix(*)
  Multiply2 : Product  OutDataTypeStr=single
  Scope : Scope  NumInputPorts=2
  低通滤波 : Subsystem  mask{fc=30, zeta=1}
      mask prompts: fc "Cut-off frequence"; zeta "Damping factor"
      mask DialogControl ParameterGroupVar Prompt: 参数
  加计-加速度估计acc_est_O_mPs2 : Outport
  wires:
  低通滤波/1(y) -> Scope/2, Delay/1
  Multiply/1 -> Scope/1, 低通滤波/1(u)  "acc_O"
  Bus Selector/1 -> Multiply/2  "<accl_B_m/s2_LPF>"
  Bus Selector1/1 -> Multiply/1  "<M_OB>"
  Rotation_Data/1 -> Bus Selector1/1
  Sensor_Data/1 -> Bus Selector/1
  Delay/1 -> 加计-加速度估计acc_est_O_mPs2/1
  Multiply2/1 -> Delay/2
  GPS_Delay/1 -> Multiply2/2
  gps_meas_valid/1 -> Multiply2/1

== system main_RI_LIEKF/State estimation/distribute CF/distribute CF/Correct/Attitude_Correction/Attitude_Correct/Subsystem2/gps_meas_acc-加速度估计 ==
  Sensor_Data : Inport
  Bus Selector1 : BusSelector  OutputSignals=GPS_Data.fixtype_gps,GPS_Data.vn_gps,GPS_Data.ve_gps,GPS_Data.vd_gps
  Compare To Constant : simulink/Logic and Bit Operations/Compare To Constant  relop=>=  const=1  OutDataTypeStr=boolean
  Detect Increase : simulink/Logic and Bit Operations/Detect Increase  vinit=0.0  OutDataTypeStr=boolean
  GPS_Meas_Acc-微分 : Subsystem  mask{fc=20, zeta=1}
      mask prompts: fc "Cut-off frequency (Hz)"; zeta "Damping factor"
  Mux : Mux  Inputs=3
  TD_baro : Subsystem
  gps_meas_acc1 : Scope  NumInputPorts=2
  gps_meas_acc2 : Scope
  gps_meas_valid : Outport
  gps_meas_acc : Outport  Port=2
  wires:
  Mux/1 -> gps_meas_acc2/1, TD_baro/1(H_baro), GPS_Meas_Acc-微分/2(gps_vel_O_mPs)
  Bus Selector1/4 -> Mux/3  "<vd_gps>"
  Sensor_Data/1 -> Bus Selector1/1
  Bus Selector1/3 -> Mux/2  "<ve_gps>"
  Compare To Constant/1 -> Detect Increase/1, GPS_Meas_Acc-微分/Enable, gps_meas_valid/1
  Bus Selector1/2 -> Mux/1  "<vn_gps>"
  Bus Selector1/1 -> Compare To Constant/1  "<fixtype_gps>"
  Detect Increase/1 -> GPS_Meas_Acc-微分/1(reset)
  GPS_Meas_Acc-微分/1(gps_acc_O_mPs2) -> gps_meas_acc1/1
  TD_baro/1(vH_baro_TD) -> gps_meas_acc1/2, gps_meas_acc/1  "vH_baro_m/s_TD"

== system main_RI_LIEKF/State estimation/distribute CF/distribute CF/Translation_estimate/Rxy_Horizontal_estimation/Rxy_kalman filter2/Vxy kalman filter/kalman ==
  note: Xk/k-1=FXk-1
      | Xk=Xk/k-1+K(Z-h(Xk/k-1))
      | K=Pk/k-1H(HPk/k-1H+Rk)-1
      | Pk/k-1=FPk-1F+GQG
      | Pk=(I-KH)Pk/k-1
  Z : Inport
  F : Inport  Port=2
  G : Inport  Port=3
  H : Inport  Port=4
  Q : Inport  Port=5
  R : Inport  Port=6
  P : Inport  Port=7
  X : Inport  Port=8
  Enable : Inport  Port=9
  Subsystem : Subsystem
  Subsystem1 : Subsystem
  POut : Outport
  XOut : Outport  Port=2
  wires:
  X/1 -> [X]
  P/1 -> [P]
  Q/1 -> [Q]
  G/1 -> [G]
  F/1 -> [F]
  Z/1 -> [Z]
  [F] -> Subsystem/1(F)
  [G] -> Subsystem/2(G)
  [Q] -> Subsystem/3(Q)
  [X] -> Subsystem/4(X)
  [P] -> Subsystem/5(P)
  Subsystem/1(Xk_k_1) -> [Xk_k_1]
  Subsystem/2(Pk_k_1) -> [Pk_k_1]
  H/1 -> Subsystem1/3(H)
  R/1 -> Subsystem1/4(R)
  Subsystem1/1(POut) -> POut/1
  Subsystem1/2(XOut) -> XOut/1
  [Xk_k_1] -> Subsystem1/1(Xkk)
  [Pk_k_1] -> Subsystem1/2(Pkk)
  Enable/1 -> Subsystem1/Enable
  [Z] -> Subsystem1/5(Z)

== system main_RI_LIEKF/State estimation/distribute CF/distribute CF/Translation_estimate/V_Horizontal_estimation/Rxy_kalman filter1/Vxy kalman filter/kalman ==
  note: Xk/k-1=FXk-1
      | Xk=Xk/k-1+K(Z-h(Xk/k-1))
      | K=Pk/k-1H(HPk/k-1H+Rk)-1
      | Pk/k-1=FPk-1F+GQG
      | Pk=(I-KH)Pk/k-1
  Z : Inport
  F : Inport  Port=2
  G : Inport  Port=3
  H : Inport  Port=4
  Q : Inport  Port=5
  R : Inport  Port=6
  P : Inport  Port=7
  X : Inport  Port=8
  Enable : Inport  Port=9
  Scope : Scope  NumInputPorts=2
  Subsystem : Subsystem
  Subsystem1 : Subsystem
  POut : Outport
  XOut : Outport  Port=2
  wires:
  [Z] -> Subsystem1/5(Z)
  Enable/1 -> Scope/1, Subsystem1/Enable
  [Pk_k_1] -> Subsystem1/2(Pkk)
  [Xk_k_1] -> Subsystem1/1(Xkk)
  Subsystem1/2(XOut) -> Scope/2, XOut/1
  Subsystem1/1(POut) -> POut/1
  R/1 -> Subsystem1/4(R)
  H/1 -> Subsystem1/3(H)
  Subsystem/2(Pk_k_1) -> [Pk_k_1]
  Subsystem/1(Xk_k_1) -> [Xk_k_1]
  [P] -> Subsystem/5(P)
  [X] -> Subsystem/4(X)
  [Q] -> Subsystem/3(Q)
  [G] -> Subsystem/2(G)
  [F] -> Subsystem/1(F)
  Z/1 -> [Z]
  F/1 -> [F]
  G/1 -> [G]
  Q/1 -> [Q]
  P/1 -> [P]
  X/1 -> [X]

== system main_RI_LIEKF/State estimation/distribute CF/distribute CF/AHRS1/Correct/Attitude_Correction/Attitude_Correct/Acc_Correct/Heading_Correct ==
  acc_est_O_mPs2 : Inport
  acc_meas_O_mPs2 : Inport  Port=2
  acc_meas_valid : Inport  Port=3
  Cross Product : FMT_Model_Lib/Math/Cross Product
  Dead Zone2 : DeadZone  LowerValue=-0.2  UpperValue=0.2
  Demux : Demux  Outputs=3
  Demux1 : Demux  Outputs=3
  Gain : Gain  Gain=INS_PARAM.HEADING_GAIN  OutDataTypeStr=single
  Gain1 : Gain  Gain=0
  Gain2 : Gain  Gain=0
  Multiply : Product
  Mux1 : Mux  Inputs=3
  Mux2 : Mux  Inputs=3
  Saturation : Saturate
  heading_correct : Outport
  wires:
  Dead Zone2/1 -> Gain/1  "test1"
  Saturation/1 -> Multiply/1
  Mux1/1 -> Cross Product/2
  Cross Product/1 -> Dead Zone2/1
  Demux/1 -> Mux1/1
  acc_meas_valid/1 -> Multiply/2
  Multiply/1 -> heading_correct/1
  Gain/1 -> Saturation/1
  acc_meas_O_mPs2/1 -> Demux/1
  Demux/2 -> Mux1/2
  Demux/3 -> Gain1/1
  Gain1/1 -> Mux1/3
  Demux1/2 -> Mux2/2
  Mux2/1 -> Cross Product/1
  Gain2/1 -> Mux2/3
  Demux1/1 -> Mux2/1
  Demux1/3 -> Gain2/1
  acc_est_O_mPs2/1 -> Demux1/1

== system main_RI_LIEKF/State estimation/distribute CF/distribute CF/AHRS1/Correct/Attitude_Correction/Attitude_Correct/Acc_Correct/Verticle_Correct ==
  acc_est_O_mPs2 : Inport
  acc_meas_O_mPs2 : Inport  Port=2
  Cross Product : FMT_Model_Lib/Math/Cross Product
  Gain : Gain  Gain=[INS_PARAM.ATT_GAIN;INS_PARAM.ATT_GAIN;0]
  Saturation : Subsystem
  Vector Normalize : FMT_Model_Lib/Math/Vector Normalize
  Vector Normalize1 : FMT_Model_Lib/Math/Vector Normalize
  vert_correct : Outport
  wires:
  Saturation/1(y) -> Gain/1
  Cross Product/1 -> Saturation/1(u)
  Vector Normalize/1 -> Cross Product/1
  acc_meas_O_mPs2/1 -> Vector Normalize1/1
  Gain/1 -> vert_correct/1
  acc_est_O_mPs2/1 -> Vector Normalize/1
  Vector Normalize1/1 -> Cross Product/2

== system main_RI_LIEKF/State estimation/distribute CF/distribute CF/AHRS1/Correct/Attitude_Correction/Attitude_Correct/Acc_Estimator/Estimate_Acc ==
  gps_meas_valid : Inport
  Sensor_Data : Inport  Port=2
  Rotation_Data : Inport  Port=3
  Bus Selector : BusSelector  OutputSignals=IMU_Data.acc_B_mPs2
  Bus Selector1 : BusSelector  OutputSignals=M_OB
  Delay : Delay  DelayLengthSource=Input port  DelayLengthUpperLimit=200
      settings: InputPortMap=u0,p1
  GPS_Delay : Constant  Value=200/INS_EXPORT.period  OutDataTypeStr=uint16
  Multiply : Product  Multiplication=Matrix(*)
  Multiply2 : Product  OutDataTypeStr=single
  Second Order LPF : FMT_Model_Lib/Filter/Second Order LPF  fc=10  zeta=0.707
  acc_est_O_mPs2 : Outport
  wires:
  Second Order LPF/1 -> Delay/1
  Multiply/1 -> Second Order LPF/1  "acc_O"
  Bus Selector/1 -> Multiply/2  "<acc_B_mPs2>"
  Bus Selector1/1 -> Multiply/1  "<M_OB>"
  Rotation_Data/1 -> Bus Selector1/1
  Sensor_Data/1 -> Bus Selector/1
  Delay/1 -> acc_est_O_mPs2/1
  Multiply2/1 -> Delay/2
  GPS_Delay/1 -> Multiply2/2
  gps_meas_valid/1 -> Multiply2/1

== system main_RI_LIEKF/State estimation/distribute CF/distribute CF/AHRS1/Correct/Attitude_Correction/Attitude_Correct/Acc_Estimator/Measure_Acc ==
  Sensor_Data : Inport
  Bus_Selection : Subsystem
  Detect Increase : simulink/Logic and Bit Operations/Detect Increase  vinit=0.0  OutDataTypeStr=boolean
  GPS_Meas_Acc : Subsystem  mask{fc=10, zeta=1}
      mask prompts: fc "Cut-off frequency (Hz)"; zeta "Damping factor"
  Valid_Check : Subsystem
  gps_meas_valid : Outport
  gps_meas_acc : Outport  Port=2
  wires:
  Valid_Check/1(gps_meas_acc_valid) -> gps_meas_valid/1, GPS_Meas_Acc/Enable, Detect Increase/1
  Detect Increase/1 -> GPS_Meas_Acc/1(reset)
  GPS_Meas_Acc/1(gps_acc_O_mPs2) -> gps_meas_acc/1
  Bus_Selection/1(gps_vel_O_mPs) -> GPS_Meas_Acc/2(gps_vel_O_mPs)
  Sensor_Data/1 -> Bus_Selection/1(Sensor_Data), Valid_Check/1(Sensor_Data)

== system main_RI_LIEKF/State estimation/distribute CF/distribute CF/Correct/Attitude_Correction/Attitude_Correct/Acc_Correct/Verticle_Correct/Normalized ==
  fb : Inport
  Add : Sum
  Constant : Constant  Value=1e-6  OutDataTypeStr=single
  Divide : Product  Inputs=*/
  Math Function : Math  Operator=magnitude^2  SignedPower=on
  Sqrt : Sqrt
  Sum of Elements : Sum  Inputs=+
  fb/g : Outport
  wires:
  Math Function/1 -> Sum of Elements/1
  Divide/1 -> fb/g/1
  Sum of Elements/1 -> Sqrt/1
  fb/1 -> Divide/1, Math Function/1
  Add/1 -> Divide/2
  Sqrt/1 -> Add/1
  Constant/1 -> Add/2

== system main_RI_LIEKF/State estimation/distribute CF/distribute CF/Correct/Attitude_Correction/Attitude_Correct/Acc_Correct/Verticle_Correct/Normalized1 ==
  fb : Inport
  Add : Sum
  Constant : Constant  Value=1e-6  OutDataTypeStr=single
  Divide : Product  Inputs=*/
  Math Function : Math  Operator=magnitude^2  SignedPower=on
  Sqrt : Sqrt
  Sum of Elements : Sum  Inputs=+
  fb/g : Outport
  wires:
  Math Function/1 -> Sum of Elements/1
  Divide/1 -> fb/g/1
  Sum of Elements/1 -> Sqrt/1
  fb/1 -> Divide/1, Math Function/1
  Add/1 -> Divide/2
  Sqrt/1 -> Add/1
  Constant/1 -> Add/2

== system main_RI_LIEKF/State estimation/distribute CF/distribute CF/Correct/Attitude_Correction/Attitude_Correct/Acc_Correct/Verticle_Correct/Saturation ==
  u : Inport
  Constant1 : Constant  Value=1e-4  OutDataTypeStr=Inherit: Inherit via back propagation
  Divide : Product  Inputs=**/
  Divide1 : Product  Inputs=*/
  Divide2 : Product  Inputs=**
  MinMax : MinMax  Function=max  Inputs=2
  Saturation : Saturate  UpperLimit=pi/2  LowerLimit=-pi/2
  Trigonometric Function : Trigonometry
  max : Constant  Value=10/180*pi  OutDataTypeStr=single
  norm : Subsystem
  y : Outport
  wires:
  Constant1/1 -> MinMax/2
  Saturation/1 -> Trigonometric Function/1
  u/1 -> norm/1(In1), Divide/1
  Trigonometric Function/1 -> Divide2/1
  Divide/1 -> y/1
  norm/1(Out1) -> Divide1/1, MinMax/1
  Divide1/1 -> Saturation/1
  Divide2/1 -> Divide/2
  max/1 -> Divide1/2, Divide2/2
  MinMax/1 -> Divide/3

== system main_RI_LIEKF/State estimation/distribute CF/distribute CF/Correct/Attitude_Correction/Attitude_Correct/Subsystem2/Estimate_Acc/低通滤波 ==
  u : Inport
  Constant : Constant  Value=0
  Discrete-Time Integrator : DiscreteIntegrator  ExternalReset=level  SampleTime=-1  ICPrevOutput=DiscIntNeverNeededParam  ICPrevScaledInput=DiscIntNeverNeededParam
  Discrete-Time Integrator1 : DiscreteIntegrator  ExternalReset=level  InitialConditionSource=external  SampleTime=-1  ICPrevOutput=DiscIntNeverNeededParam  ICPrevScaledInput=DiscIntNeverNeededParam
  Gain : Gain  Gain=(2*pi*fc)^2
  Gain1 : Gain  Gain=2*zeta*(2*pi*fc)
  Sum : Sum  Inputs=|+-
  Sum1 : Sum  Inputs=|+-
  y : Outport
  wires:
  Sum/1 -> Gain/1
  Discrete-Time Integrator1/1 -> y/1, Sum/2
  Discrete-Time Integrator/1 -> Gain1/1, Discrete-Time Integrator1/1
  Sum1/1 -> Discrete-Time Integrator/1
  Constant/1 -> Discrete-Time Integrator1/2, Discrete-Time Integrator/2
  u/1 -> Discrete-Time Integrator1/3, Sum/1
  Gain1/1 -> Sum1/2
  Gain/1 -> Sum1/1

== system main_RI_LIEKF/State estimation/distribute CF/distribute CF/Correct/Attitude_Correction/Attitude_Correct/Subsystem2/gps_meas_acc-加速度估计/GPS_Meas_Acc-微分 ==
  reset : Inport
  gps_vel_O_mPs : Inport  Port=2
  Enable : EnablePort  StatesWhenEnabling=reset
  Integrator : DiscreteIntegrator  ExternalReset=level  SampleTime=-1  ICPrevOutput=DiscIntNeverNeededParam  ICPrevScaledInput=DiscIntNeverNeededParam
  Integrator1 : DiscreteIntegrator  ExternalReset=level  InitialConditionSource=external  SampleTime=-1  ICPrevOutput=DiscIntNeverNeededParam  ICPrevScaledInput=DiscIntNeverNeededParam
  Sum : Sum  Inputs=|++
  Sum1 : Sum  Inputs=|+-
  gain : Gain  Gain=2*zeta*fc
  gain1 : Gain  Gain=fc^2
  gps_acc_O_mPs2 : Outport
  wires:
  Integrator1/1 -> Sum1/2
  Integrator/1 -> gps_acc_O_mPs2/1, Sum/2
  reset/1 -> Integrator1/2, Integrator/2
  gain/1 -> Sum/1
  Sum1/1 -> gain/1, gain1/1
  Sum/1 -> Integrator1/1
  gps_vel_O_mPs/1 -> Sum1/1, Integrator1/3
  gain1/1 -> Integrator/1

== system main_RI_LIEKF/State estimation/distribute CF/distribute CF/Correct/Attitude_Correction/Attitude_Correct/Subsystem2/gps_meas_acc-加速度估计/TD_baro ==
  H_baro : Inport
  Demux : Demux  Outputs=3
  Mux : Mux  Inputs=3
  Subsystem : Subsystem
  Subsystem1 : Subsystem
  Subsystem2 : Subsystem
  vH_baro_TD : Outport
  wires:
  Demux/2 -> Subsystem1/1(In1)
  H_baro/1 -> Demux/1
  Demux/1 -> Subsystem/1(In1)
  Demux/3 -> Subsystem2/1(In1)
  Subsystem/1(u2) -> Mux/1
  Subsystem1/1(u2) -> Mux/2
  Subsystem2/1(u2) -> Mux/3
  Mux/1 -> vH_baro_TD/1

== system main_RI_LIEKF/State estimation/distribute CF/distribute CF/Translation_estimate/Rxy_Horizontal_estimation/Rxy_kalman filter2/Vxy kalman filter/kalman/Subsystem ==
  F : Inport
  G : Inport  Port=2
  Q : Inport  Port=3
  X : Inport  Port=4
  P : Inport  Port=5
  Add : Sum
  Math Function3 : Math  Operator=transpose  SignedPower=on
  Math Function4 : Math  Operator=transpose  SignedPower=on
  MatrixMultiply : Product  Multiplication=Matrix(*)
  MatrixMultiply1 : Product  Inputs=3  Multiplication=Matrix(*)
  MatrixMultiply8 : Product  Inputs=3  Multiplication=Matrix(*)
  Xk_k_1 : Outport
  Pk_k_1 : Outport  Port=2
  wires:
  Math Function4/1 -> MatrixMultiply8/3
  [Q] -> MatrixMultiply8/2
  MatrixMultiply/1 -> [Xk_k_1]
  MatrixMultiply1/1 -> Add/1
  [F] -> Math Function3/1
  Math Function3/1 -> MatrixMultiply1/3
  [P] -> MatrixMultiply1/2
  [F] -> MatrixMultiply1/1
  Add/1 -> [Pk_k_1]
  [G] -> MatrixMultiply8/1
  MatrixMultiply8/1 -> Add/2
  [X] -> MatrixMultiply/2
  [G] -> Math Function4/1
  [F] -> MatrixMultiply/1
  F/1 -> [F]
  G/1 -> [G]
  Q/1 -> [Q]
  X/1 -> [X]
  P/1 -> [P]
  [Xk_k_1] -> Xk_k_1/1
  [Pk_k_1] -> Pk_k_1/1

== system main_RI_LIEKF/State estimation/distribute CF/distribute CF/Translation_estimate/Rxy_Horizontal_estimation/Rxy_kalman filter2/Vxy kalman filter/kalman/Subsystem1 ==
  note: 计算卡尔曼增益Kk
  Xkk : Inport
  Pkk : Inport  Port=2
  H : Inport  Port=3
  R : Inport  Port=4
  Z : Inport  Port=5
  Enable : EnablePort
  Add2 : Sum
  Add3 : Sum  Inputs=+-
  Add4 : Sum  Inputs=+-
  Add5 : Sum
  Constant : Constant  Value=eye(4)  OutDataTypeStr=single
  LDL Solver1 : dspsolvers/LDL Solver  errmode=Warning
      settings: RTWMemSecFuncInitTerm=Default  RTWMemSecFuncExecute=Default  RTWMemSecDataConstants=Default  RTWMemSecDataInternal=Default  RTWMemSecDataParameters=Default
  Math Function5 : Math  Operator=transpose  SignedPower=on
  Math Function6 : Math  Operator=transpose  SignedPower=on
  MatrixMultiply{4..7,9..10} (6 alike) : Product  Multiplication=Matrix(*)
  Scope : Scope
  POut : Outport
  XOut : Outport  Port=2
  wires:
  MatrixMultiply9/1 -> Add3/2
  MatrixMultiply7/1 -> POut/1
  [H] -> MatrixMultiply10/1
  Add3/1 -> MatrixMultiply4/2
  Math Function5/1 -> MatrixMultiply5/2
  Math Function6/1 -> Scope/1, [Kk]
  Add4/1 -> MatrixMultiply7/1
  MatrixMultiply4/1 -> Add2/2
  [Kk] -> MatrixMultiply4/1
  [Z] -> Add3/1
  MatrixMultiply10/1 -> MatrixMultiply5/1, LDL Solver1/2
  MatrixMultiply5/1 -> Add5/1
  LDL Solver1/1 -> Math Function6/1
  [H] -> Math Function5/1
  [Pk_k_1] -> MatrixMultiply10/2
  [R] -> Add5/2
  Constant/1 -> Add4/1
  [Kk] -> MatrixMultiply6/1
  [Xk_k_1] -> Add2/1
  [H] -> MatrixMultiply6/2
  [H] -> MatrixMultiply9/1
  [Xk_k_1] -> MatrixMultiply9/2
  [Pk_k_1] -> MatrixMultiply7/2
  R/1 -> [R]
  Add5/1 -> LDL Solver1/1
  MatrixMultiply6/1 -> Add4/2
  H/1 -> [H]
  Add2/1 -> XOut/1
  Xkk/1 -> [Xk_k_1]
  Z/1 -> [Z]
  Pkk/1 -> [Pk_k_1]
